simulink model "TapDL_resistor"  (R2020b)
settings: Solver=FixedStepAuto  StartTime=0.0  StopTime=TFinal  RelTol=1e-3
undefined symbols (not defined in the file or in its folder): coupling, decay_rate, n, nodes, sample_time
libraries: simrfV2util1 x6, simrfV2_lib x2, simrfV2elements x2, simulink x1
settings Model: Creator=tg847  LastModifiedBy=tian

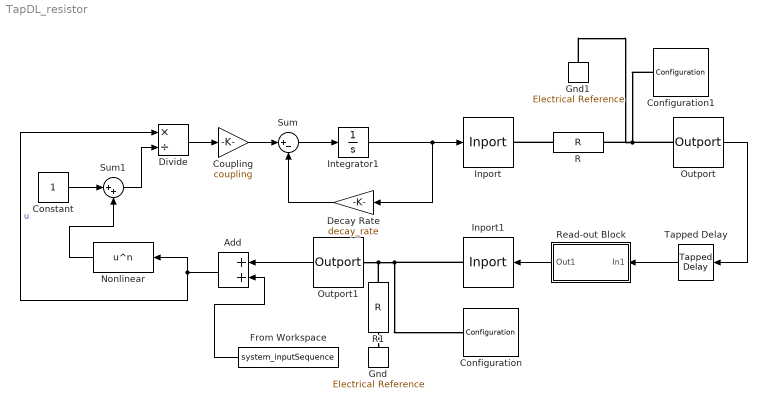
== system TapDL_resistor ==
  Add : Sum
  Configuration : simrfV2util1/Configuration  AutoFreq=on  Tones=[0] Hz  Harmonics=[1]  NormalizeCarrierPower=on  SolverType=Auto  UseCCode=on  StepSize=0.06/10 s  AddNoise=off  defaultRNG=on  Seed=0  Temperature=290.0 K  SolverDelFlag=0  AbsTol=1e-6  RelTol=1e-3  MaxIter=10  ErrorEstimationType=2-norm over all variables  EnableInterpFilter=off  HiddenFIRfilterControllerParam=on  SmallSignalApprox=off  AllSimFreqs=on  SimFreqs=[] Hz  SimFreqsInternal=[]  SamplesPerFrame=1
      settings: SourceProductBaseCode=RB
  Configuration1 : simrfV2util1/Configuration  AutoFreq=on  Tones=[0] Hz  Harmonics=[1]  NormalizeCarrierPower=on  SolverType=Auto  UseCCode=on  StepSize=0.06/10 s  AddNoise=off  defaultRNG=on  Seed=0  Temperature=290.0 K  SolverDelFlag=0  AbsTol=1e-6  RelTol=1e-3  MaxIter=10  ErrorEstimationType=2-norm over all variables  EnableInterpFilter=off  HiddenFIRfilterControllerParam=on  SmallSignalApprox=off  AllSimFreqs=on  SimFreqs=[] Hz  SimFreqsInternal=[]  SamplesPerFrame=1
      settings: SourceProductBaseCode=RB
  Constant : Constant
  Coupling : Gain  Gain=coupling
      mask Display: fprintf("%c", 946)
  "Decay Rate " : Gain  Gain=decay_rate
      mask Display: fprintf("%c", 947)
  Divide : Product  Inputs=*/
  From Workspace : FromWorkspace  VariableName=system_inputSequence
  Gnd : simrfV2_lib/Elements/Electrical Reference
      settings: SourceProductBaseCode=RB  InternalSimscapePortConfiguration="{\"Bottom\":[],\"Left\":[{\"id\":\"V\",\"label\":\"\",\"type\":\"foundation.rf.circuitenvelope\"}],\"Right\":[],\"Top\":[]}"
  Gnd1 : simrfV2_lib/Elements/Electrical Reference
      settings: SourceProductBaseCode=RB  InternalSimscapePortConfiguration="{\"Bottom\":[],\"Left\":[{\"id\":\"V\",\"label\":\"\",\"type\":\"foundation.rf.circuitenvelope\"}],\"Right\":[],\"Top\":[]}"
  Inport : simrfV2util1/Inport  SimulinkInputSignalType=Ideal voltage  CarrierFreq=0 Hz  ZS=0  InternalGrounding=on
      settings: SourceProductBaseCode=RB
  Inport1 : simrfV2util1/Inport  SimulinkInputSignalType=Ideal voltage  CarrierFreq=0 Hz  ZS=0  InternalGrounding=on
      settings: SourceProductBaseCode=RB
  Integrator1 : Integrator  IgnoreLimit=on
  Nonlinear : Fcn  Expr=u^n
  Outport : simrfV2util1/Outport  SensorType=Ideal voltage  OutputFormat=Real Passband  CarrierFreq=0 Hz  ZL=Inf  InternalGrounding=on  StepSize=0.006 s  AutoStep=on
      settings: SourceProductBaseCode=RB
  Outport1 : simrfV2util1/Outport  SensorType=Ideal voltage  OutputFormat=Real Passband  CarrierFreq=0 Hz  ZL=Inf  InternalGrounding=on  StepSize=0.006 s  AutoStep=on
      settings: SourceProductBaseCode=RB
  R : simrfV2elements/R  classname=resistor  Resistance=800 Ohm  AddNoise=off
      settings: SourceProductBaseCode=RB
  R1 : simrfV2elements/R  classname=resistor  Resistance=800 Ohm  AddNoise=off
      settings: SourceProductBaseCode=RB
  Read-out Block : Subsystem
  Sum : Sum  Inputs=|+-
  Sum1 : Sum  Inputs=|++
  Tapped Delay : simulink/Discrete/Tapped Delay  vinit=0.0  samptime=theta  NumDelays=nodes  DelayOrder=Oldest  includeCurrent=off
  wires:
  Add/1 -> Divide/1, Nonlinear/1  "u"
  Coupling/1 -> Sum/1
  Sum1/1 -> Divide/2
  From Workspace/1 -> Add/2
  Divide/1 -> Coupling/1
  Nonlinear/1 -> Sum1/2
  Constant/1 -> Sum1/1
  Sum/1 -> Integrator1/1
  Integrator1/1 -> Inport/1, "Decay Rate "/1
  "Decay Rate "/1 -> Sum/2
  Tapped Delay/1 -> Read-out Block/1(In1)
  Outport/1 -> Tapped Delay/1
  Outport1/1 -> Add/1
  Read-out Block/1(Out1) -> Inport1/1
  connections:
  R/LConn1 -- Inport/RConn1
  Outport/LConn1 -- Gnd1/LConn1 -- R/RConn1 -- Configuration1/LConn1
  Outport1/LConn1 -- R1/RConn1 -- Inport1/RConn1 -- Configuration/LConn1
  R1/LConn1 -- Gnd/LConn1

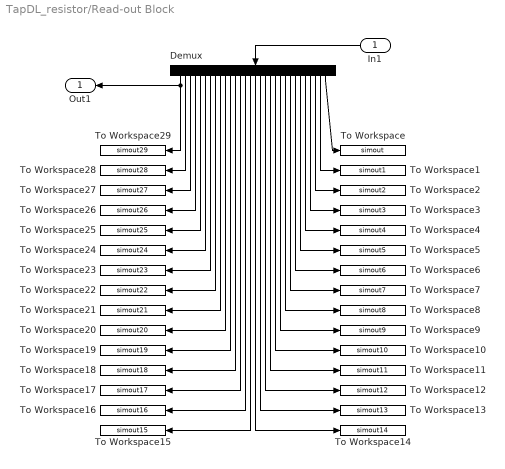
== system TapDL_resistor/Read-out Block ==
  In1 : Inport
  Demux : Demux  Outputs=30
      settings: DisplayOption=none
  To Workspace : ToWorkspace  VariableName=simout  SampleTime=sample_time
  To Workspace1 : ToWorkspace  VariableName=simout1  SampleTime=sample_time
  To Workspace10 : ToWorkspace  VariableName=simout10  SampleTime=sample_time
  To Workspace11 : ToWorkspace  VariableName=simout11  SampleTime=sample_time
  To Workspace12 : ToWorkspace  VariableName=simout12  SampleTime=sample_time
  To Workspace13 : ToWorkspace  VariableName=simout13  SampleTime=sample_time
  To Workspace14 : ToWorkspace  VariableName=simout14  SampleTime=sample_time
  To Workspace15 : ToWorkspace  VariableName=simout15  SampleTime=sample_time
  To Workspace16 : ToWorkspace  VariableName=simout16  SampleTime=sample_time
  To Workspace17 : ToWorkspace  VariableName=simout17  SampleTime=sample_time
  To Workspace18 : ToWorkspace  VariableName=simout18  SampleTime=sample_time
  To Workspace19 : ToWorkspace  VariableName=simout19  SampleTime=sample_time
  To Workspace2 : ToWorkspace  VariableName=simout2  SampleTime=sample_time
  To Workspace20 : ToWorkspace  VariableName=simout20  SampleTime=sample_time
  To Workspace21 : ToWorkspace  VariableName=simout21  SampleTime=sample_time
  To Workspace22 : ToWorkspace  VariableName=simout22  SampleTime=sample_time
  To Workspace23 : ToWorkspace  VariableName=simout23  SampleTime=sample_time
  To Workspace24 : ToWorkspace  VariableName=simout24  SampleTime=sample_time
  To Workspace25 : ToWorkspace  VariableName=simout25  SampleTime=sample_time
  To Workspace26 : ToWorkspace  VariableName=simout26  SampleTime=sample_time
  To Workspace27 : ToWorkspace  VariableName=simout27  SampleTime=sample_time
  To Workspace28 : ToWorkspace  VariableName=simout28  SampleTime=sample_time
  To Workspace29 : ToWorkspace  VariableName=simout29  SampleTime=sample_time
  To Workspace3 : ToWorkspace  VariableName=simout3  SampleTime=sample_time
  To Workspace4 : ToWorkspace  VariableName=simout4  SampleTime=sample_time
  To Workspace5 : ToWorkspace  VariableName=simout5  SampleTime=sample_time
  To Workspace6 : ToWorkspace  VariableName=simout6  SampleTime=sample_time
  To Workspace7 : ToWorkspace  VariableName=simout7  SampleTime=sample_time
  To Workspace8 : ToWorkspace  VariableName=simout8  SampleTime=sample_time
  To Workspace9 : ToWorkspace  VariableName=simout9  SampleTime=sample_time
  Out1 : Outport
  wires:
  Demux/17 -> To Workspace13/1
  Demux/27 -> To Workspace3/1
  Demux/12 -> To Workspace18/1
  Demux/9 -> To Workspace21/1
  Demux/21 -> To Workspace9/1
  Demux/3 -> To Workspace27/1
  Demux/14 -> To Workspace16/1
  Demux/26 -> To Workspace4/1
  Demux/2 -> To Workspace28/1
  Demux/18 -> To Workspace12/1
  Demux/28 -> To Workspace2/1
  Demux/5 -> To Workspace25/1
  Demux/19 -> To Workspace11/1
  Demux/22 -> To Workspace8/1
  Demux/13 -> To Workspace17/1
  Demux/8 -> To Workspace22/1
  Demux/15 -> To Workspace15/1
  Demux/1 -> Out1/1, To Workspace29/1
  Demux/16 -> To Workspace14/1
  Demux/29 -> To Workspace1/1
  Demux/25 -> To Workspace5/1
  In1/1 -> Demux/1
  Demux/7 -> To Workspace23/1
  Demux/20 -> To Workspace10/1
  Demux/6 -> To Workspace24/1
  Demux/30 -> To Workspace/1
  Demux/24 -> To Workspace6/1
  Demux/10 -> To Workspace20/1
  Demux/4 -> To Workspace26/1
  Demux/23 -> To Workspace7/1
  Demux/11 -> To Workspace19/1
